simulink model "Controllo_postura_uniciclo"  (R2021b)
settings: Solver=ode1be  StartTime=0.0  StopTime=20  FixedStep=0.025  RelTol=1e-3
values from neighbouring files (symbols this model uses):
  Klya = [k1, k2, l2]    [init.m]
  q0 = [-10; -10; -pi]    [init.m]
settings Model: Creator=vince  LastModifiedBy=vince

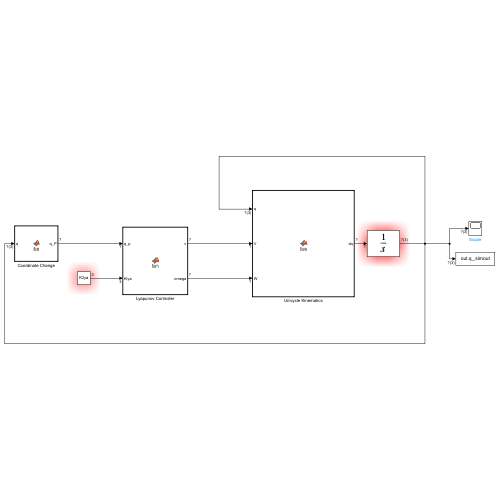
[thumbnail: Simulink's stored preview of the top-level diagram]
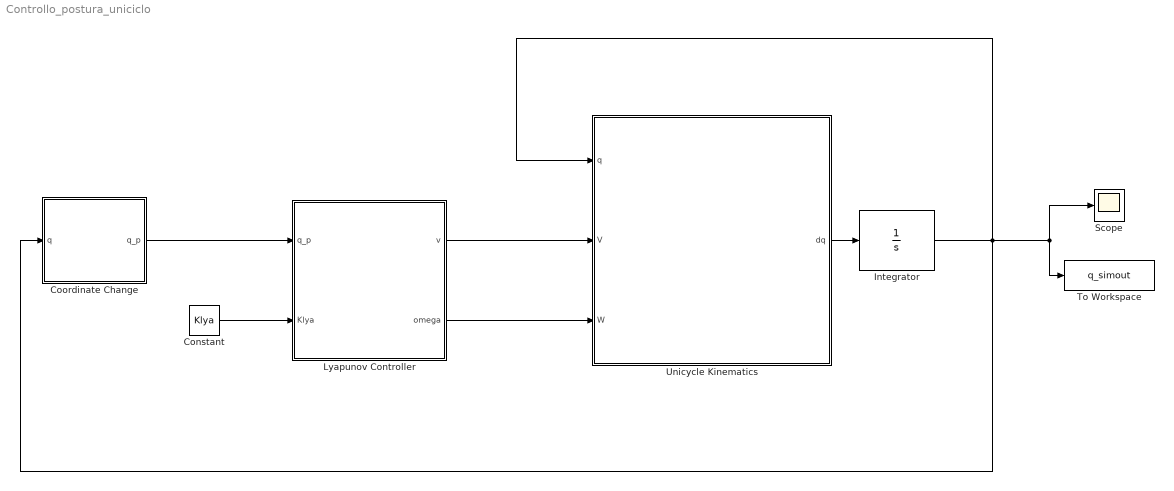
== system Controllo_postura_uniciclo ==
  Constant : Constant  Value=Klya
  Coordinate Change : MATLAB Function  TreatAsAtomicUnit=on
  Integrator : Integrator  InitialCondition=q0
  Lyapunov Controller : MATLAB Function  TreatAsAtomicUnit=on
  Scope : Scope
  To Workspace : ToWorkspace  VariableName=q_simout  SaveFormat=Timeseries  SampleTime=-1
  Unicycle Kinematics : MATLAB Function  TreatAsAtomicUnit=on
  wires:
  Coordinate Change/1(q_p) -> Lyapunov Controller/1(q_p)
  Lyapunov Controller/1(v) -> Unicycle Kinematics/2(V)
  Integrator/1 -> Scope/1, To Workspace/1, Unicycle Kinematics/1(q), Coordinate Change/1(q)
  Unicycle Kinematics/1(dq) -> Integrator/1
  Lyapunov Controller/2(omega) -> Unicycle Kinematics/3(W)
  Constant/1 -> Lyapunov Controller/2(Klya)

== matlab function Controllo_postura_uniciclo/Lyapunov Controller ==
  data: q_p input; v output; Klya input; omega output
function [v, omega] = fcn(q_p, Klya)

rho = q_p(1); phi = q_p(2); alpha = q_p(3);

% parametri 

k1 = Klya(1); k2 = Klya(2); lambda2 = Klya(3);

% control
v = rho*k1*cos(alpha);

% se x tende a 0 allora sen(x)/x = 1
if alpha <= 0.0001
    omega = k1*cos(alpha)*(alpha+lambda2*phi)+k2*alpha;
else
    omega = k1*(sin(alpha)/alpha)*cos(alpha)*(alpha+lambda2*phi)+k2*alpha;
end

== matlab function Controllo_postura_uniciclo/Coordinate Change ==
  data: q input; q_p output
function q_p = fcn(q)
 
x = q(1); y = q(2); th = q(3);
rho = sqrt(x^2 + y^2);
phi = atan2(y,x)+pi;
alpha = phi - th;

% Angles normalization
while (phi >= pi)
    phi = phi - 2*pi;
end
while (phi < -pi)
    phi = phi + 2*pi;
end

q_p = [rho; phi; alpha];

== matlab function Controllo_postura_uniciclo/Unicycle Kinematics ==
  data: q input; dq output; V input; W input
function dq = fcn(q, V, W)

x = q(1); y = q(2); th = q(3);

dx = V * cos(th);
dy = V * sin(th);
dth = W;

dq = [dx; dy; dth];
